simulink model "UPS_3level_Ttype_Inverter_simplified_ctrl_v3"  (R2012b)
settings: Solver=ode4  StartTime=0.0  StopTime=Tfinal  FixedStep=Ts  MaxStep=1e-5  RelTol=1e-3
values from neighbouring files (symbols this model uses):
  FACT = 1    [simulate_steady_state.m]    (also in simulate_transient.m)
undefined symbols (not defined in the file or in its folder): ADC, CTRL, DiscIntNeverNeededParam, PR, S, Ts, UPS, Vd, VSI
libraries: powerlib x113, simulink_extras x11, powerlib_extras x11, simulink x3
(part 3 of 3)

== system UPS_3level_Ttype_Inverter_simplified_ctrl_v3/Output Inverter Control System SRF(dq0) - SPWM /SPWM (Treg)2/controller ph a3/vCf reference ==
  cos* sin* : Inport
  vs* [V] : Inport  Port=2
  Product3 : Product  RndMeth=Zero
  vCf_ref [V] : Outport
  wires:
  vs* [V]/1 -> Product3/2
  Product3/1 -> vCf_ref [V]/1
  cos* sin*/1 -> Product3/1
